simulink model "ball_bounce"  (R2020a)
settings: Solver=VariableStepAuto  StartTime=0.0  StopTime=50.0  RelTol=1e-3
undefined symbols (not defined in the file): out
settings Model: Creator=admin  LastModifiedBy=admin

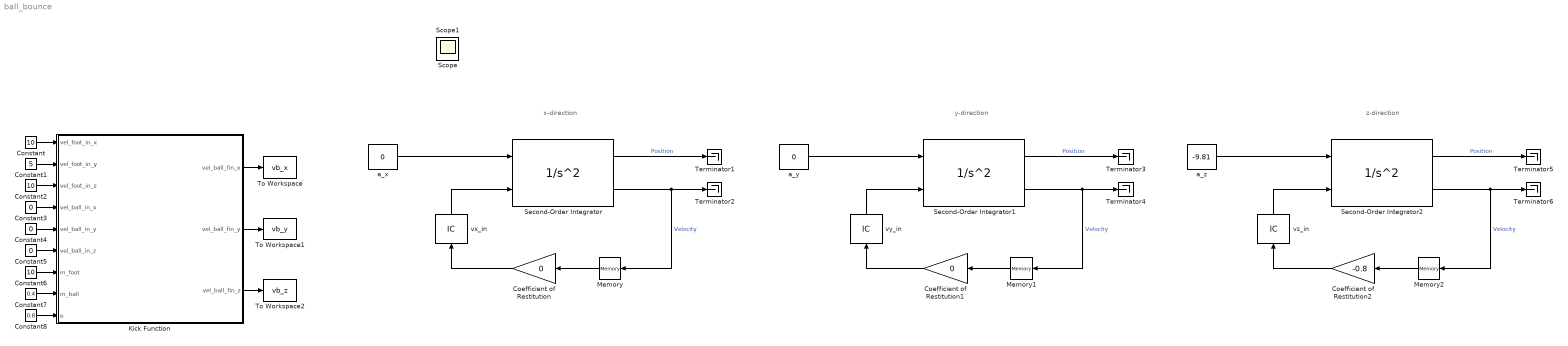
== system ball_bounce ==
  note: x-direction
  note: y-direction
  note: z-direction
  Coefficient of Restitution : Gain  Gain=0
  Coefficient of Restitution1 : Gain  Gain=0
  Coefficient of Restitution2 : Gain  Gain=-0.8
  Constant : Constant  Value=10
  Constant1 : Constant  Value=5
  Constant2 : Constant  Value=10
  Constant3 : Constant  Value=0
  Constant4 : Constant  Value=0
  Constant5 : Constant  Value=0
  Constant6 : Constant  Value=10
  Constant7 : Constant  Value=0.4
  Constant8 : Constant  Value=0.8
  Kick Function : MATLAB Function  TreatAsAtomicUnit=on
  Memory : Memory
  Memory1 : Memory
  Memory2 : Memory
  Second-Order Integrator : SecondOrderIntegrator  ICX=10.0  LimitX=on  LowerLimitX=0.0  StateNameX='Position'  ICSourceDXDT=external  StateNameDXDT='Velocity'  ReinitDXDTwhenXreachesSaturation=on
  Second-Order Integrator1 : SecondOrderIntegrator  ICX=10.0  LimitX=on  LowerLimitX=0.0  StateNameX='Position'  ICSourceDXDT=external  StateNameDXDT='Velocity'  ReinitDXDTwhenXreachesSaturation=on
  Second-Order Integrator2 : SecondOrderIntegrator  ICX=10.0  LimitX=on  LowerLimitX=0.0  StateNameX='Position'  ICSourceDXDT=external  StateNameDXDT='Velocity'  ReinitDXDTwhenXreachesSaturation=on
  Terminator{1..6} (6 alike) : Terminator
  To Workspace : ToWorkspace  VariableName=vb_x  SaveFormat=Timeseries  SampleTime=-1
  To Workspace1 : ToWorkspace  VariableName=vb_y  SaveFormat=Timeseries  SampleTime=-1
  To Workspace2 : ToWorkspace  VariableName=vb_z  SaveFormat=Timeseries  SampleTime=-1
  a_x : Constant  Value=0  OutDataTypeStr=double
  a_y : Constant  Value=0  OutDataTypeStr=double
  a_z : Constant  Value=-9.81  OutDataTypeStr=double
  "vx_in " : InitialCondition  Value=out.vb_x
  vy_in : InitialCondition  Value=out.vb_y
  vz_in : InitialCondition  Value=out.vb_z
  Scope : Scope
  Scope1 : Scope
  wires:
  Coefficient of Restitution1/1 -> vy_in/1
  vy_in/1 -> Second-Order Integrator1/2
  a_y/1 -> Second-Order Integrator1/1
  Second-Order Integrator1/2 -> Memory1/1, Terminator4/1  "Velocity"
  Second-Order Integrator1/1 -> Terminator3/1  "Position"
  Memory1/1 -> Coefficient of Restitution1/1
  a_x/1 -> Second-Order Integrator/1
  Coefficient of Restitution/1 -> "vx_in "/1
  Second-Order Integrator/2 -> Memory/1, Terminator2/1  "Velocity"
  Second-Order Integrator/1 -> Terminator1/1  "Position"
  Memory/1 -> Coefficient of Restitution/1
  "vx_in "/1 -> Second-Order Integrator/2
  Memory2/1 -> Coefficient of Restitution2/1
  a_z/1 -> Second-Order Integrator2/1
  Second-Order Integrator2/2 -> Memory2/1, Terminator6/1  "Velocity"
  Coefficient of Restitution2/1 -> vz_in/1
  Second-Order Integrator2/1 -> Terminator5/1  "Position"
  vz_in/1 -> Second-Order Integrator2/2
  Constant/1 -> Kick Function/1(vel_foot_in_x)
  Constant1/1 -> Kick Function/2(vel_foot_in_y)
  Constant2/1 -> Kick Function/3(vel_foot_in_z)
  Constant3/1 -> Kick Function/4(vel_ball_in_x)
  Constant4/1 -> Kick Function/5(vel_ball_in_y)
  Constant5/1 -> Kick Function/6(vel_ball_in_z)
  Constant6/1 -> Kick Function/7(m_foot)
  Constant7/1 -> Kick Function/8(m_ball)
  Constant8/1 -> Kick Function/9(e)
  Kick Function/1(vel_ball_fin_x) -> To Workspace/1
  Kick Function/2(vel_ball_fin_y) -> To Workspace1/1
  Kick Function/3(vel_ball_fin_z) -> To Workspace2/1

== matlab function ball_bounce/Kick Function ==
  data: vel_foot_in_x input; vel_ball_fin_x output; vel_foot_in_y input; vel_foot_in_z input; vel_ball_in_x input; vel_ball_in_y input; vel_ball_in_z input; m_foot input; m_ball input; e input; vel_ball_fin_y output; vel_ball_fin_z output
function [vel_ball_fin_x, vel_ball_fin_y, vel_ball_fin_z] = kick(vel_foot_in_x, vel_foot_in_y, vel_foot_in_z, vel_ball_in_x, vel_ball_in_y, vel_ball_in_z, m_foot, m_ball, e)
vel_ball_fin_x = (((vel_foot_in_x * m_foot * (1 + e)) + (vel_ball_in_x * (m_ball - e * m_foot)))/ (m_foot + m_ball));
vel_ball_fin_y = (((vel_foot_in_y * m_foot * (1 + e)) + (vel_ball_in_y * (m_ball - e * m_foot)))/ (m_foot + m_ball));
vel_ball_fin_z = (((vel_foot_in_z * m_foot * (1 + e)) + (vel_ball_in_z * (m_ball - e * m_foot)))/ (m_foot + m_ball));
end
